simulink subsystem "April_Tag_Errors"  (R2023b)
settings: Solver=VariableStepAuto  StartTime=0.0  StopTime=10.0  RelTol=1e-3
undefined symbols (not defined in the file): AT_Tag_11_Yaw_Offset, AT_Tag_12_Yaw_Offset, AT_Tag_13_Coordinate_Y, AT_Tag_13_Yaw_Offset, AT_Tag_14_Coordinate_Y, AT_Tag_14_Yaw_Offset, AT_Tag_15_Yaw_Offset, AT_Tag_16_Yaw_Offset, AT_Tag_4_Yaw_Offset, AT_Tag_5_Coordinate_X, AT_Tag_5_Yaw_Offset, AT_Tag_6_Coordinate_X, AT_Tag_6_Yaw_Offset, AT_Tag_7_Yaw_Offset, KF_Vision_Ambiguity_Thresh
libraries: simulink x1
settings Model: Creator=ander  LastModifiedBy=ander

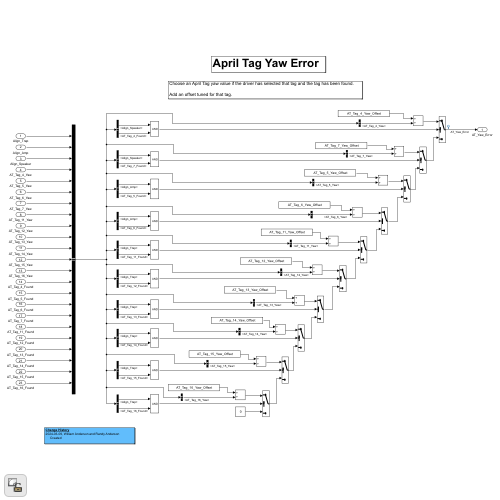
[thumbnail: Simulink's stored preview of the top-level diagram]
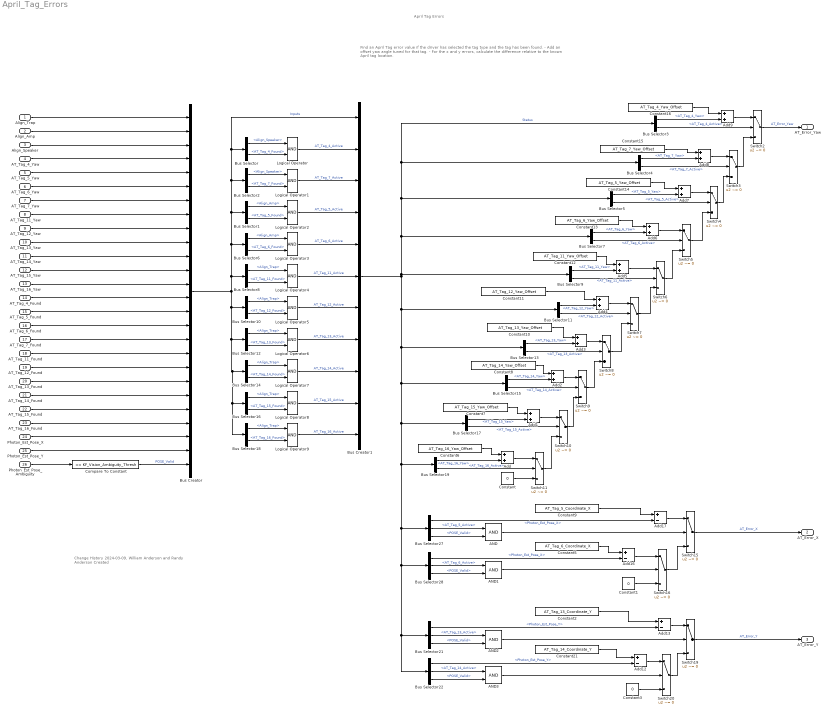
== system April_Tag_Errors ==
  note: Find an April Tag error value if the driver has selected the tag type and the tag has been found.
      | - Add an offset yaw angle tuned for that tag.
      | - For the x and y errors, calculate the difference relative to the known April tag location.
  note: Change History
      | 2024-03-09, William Anderson and Randy Anderson
      | Created
  note: April Tag Errors
  Align_Trap : Inport
  Align_Amp : Inport  Port=2
  Align_Speaker : Inport  Port=3
  AT_Tag_4_Yaw : Inport  Port=4
  AT_Tag_5_Yaw : Inport  Port=5
  AT_Tag_6_Yaw : Inport  Port=6
  AT_Tag_7_Yaw : Inport  Port=7
  AT_Tag_11_Yaw : Inport  Port=8
  AT_Tag_12_Yaw : Inport  Port=9
  AT_Tag_13_Yaw : Inport  Port=10
  AT_Tag_14_Yaw : Inport  Port=11
  AT_Tag_15_Yaw : Inport  Port=12
  AT_Tag_16_Yaw : Inport  Port=13
  AT_Tag_4_Found : Inport  Port=14
  AT_Tag_5_Found : Inport  Port=15
  AT_Tag_6_Found : Inport  Port=16
  AT_Tag_7_Found : Inport  Port=17
  AT_Tag_11_Found : Inport  Port=18
  AT_Tag_12_Found : Inport  Port=19
  AT_Tag_13_Found : Inport  Port=20
  AT_Tag_14_Found : Inport  Port=21
  AT_Tag_15_Found : Inport  Port=22
  AT_Tag_16_Found : Inport  Port=23
  Photon_Est_Pose_X : Inport  Port=24
  Photon_Est_Pose_Y : Inport  Port=25
  Photon_Est_Pose_Ambiguity : Inport  Port=26
  AND{,1..3} (4 alike) : Logic  AllPortsSameDT=off  OutDataTypeStr=boolean
  Add{,1..9} (10 alike) : Sum
  Add{12..13,16..17} (4 alike) : Sum  Inputs=+-
  Bus Creator : BusCreator  Inputs=26
  Bus Creator1 : BusCreator  Inputs=11
  Bus Selector : BusSelector  OutputSignals=Align_Speaker,AT_Tag_4_Found
  Bus Selector1 : BusSelector  OutputSignals=Align_Amp,AT_Tag_5_Found
  Bus Selector10 : BusSelector  OutputSignals=Align_Trap,AT_Tag_12_Found
  Bus Selector11 : BusSelector  OutputSignals=Inputs.AT_Tag_12_Yaw,AT_Tag_12_Active
  Bus Selector12 : BusSelector  OutputSignals=Align_Trap,AT_Tag_13_Found
  Bus Selector13 : BusSelector  OutputSignals=Inputs.AT_Tag_13_Yaw,AT_Tag_13_Active
  Bus Selector14 : BusSelector  OutputSignals=Align_Trap,AT_Tag_14_Found
  Bus Selector15 : BusSelector  OutputSignals=Inputs.AT_Tag_14_Yaw,AT_Tag_14_Active
  Bus Selector16 : BusSelector  OutputSignals=Align_Trap,AT_Tag_15_Found
  Bus Selector17 : BusSelector  OutputSignals=Inputs.AT_Tag_15_Yaw,AT_Tag_15_Active
  Bus Selector18 : BusSelector  OutputSignals=Align_Trap,AT_Tag_16_Found
  Bus Selector19 : BusSelector  OutputSignals=Inputs.AT_Tag_16_Yaw,AT_Tag_16_Active
  Bus Selector2 : BusSelector  OutputSignals=Align_Speaker,AT_Tag_7_Found
  Bus Selector21 : BusSelector  OutputSignals=Inputs.Photon_Est_Pose_Y,AT_Tag_13_Active,Inputs.POSE_Valid
  Bus Selector22 : BusSelector  OutputSignals=Inputs.Photon_Est_Pose_Y,AT_Tag_14_Active,Inputs.POSE_Valid
  Bus Selector27 : BusSelector  OutputSignals=Inputs.Photon_Est_Pose_X,AT_Tag_5_Active,Inputs.POSE_Valid
  Bus Selector28 : BusSelector  OutputSignals=Inputs.Photon_Est_Pose_X,AT_Tag_6_Active,Inputs.POSE_Valid
  Bus Selector3 : BusSelector  OutputSignals=Inputs.AT_Tag_4_Yaw,AT_Tag_4_Active
  Bus Selector4 : BusSelector  OutputSignals=Inputs.AT_Tag_7_Yaw,AT_Tag_7_Active
  Bus Selector5 : BusSelector  OutputSignals=Inputs.AT_Tag_5_Yaw,AT_Tag_5_Active
  Bus Selector6 : BusSelector  OutputSignals=Align_Amp,AT_Tag_6_Found
  Bus Selector7 : BusSelector  OutputSignals=Inputs.AT_Tag_6_Yaw,AT_Tag_6_Active
  Bus Selector8 : BusSelector  OutputSignals=Align_Trap,AT_Tag_11_Found
  Bus Selector9 : BusSelector  OutputSignals=Inputs.AT_Tag_11_Yaw,AT_Tag_11_Active
  Compare To Constant : simulink/Logic and Bit Operations/Compare To Constant  relop=<=  const=KF_Vision_Ambiguity_Thresh  OutDataTypeStr=boolean
  Constant : Constant  Value=0
  Constant1 : Constant  Value=0
  Constant10 : Constant  Value=AT_Tag_13_Yaw_Offset
  Constant11 : Constant  Value=AT_Tag_12_Yaw_Offset
  Constant12 : Constant  Value=AT_Tag_11_Yaw_Offset
  Constant13 : Constant  Value=AT_Tag_6_Yaw_Offset
  Constant14 : Constant  Value=AT_Tag_5_Yaw_Offset
  Constant15 : Constant  Value=AT_Tag_7_Yaw_Offset
  Constant16 : Constant  Value=AT_Tag_4_Yaw_Offset
  Constant2 : Constant  Value=AT_Tag_13_Coordinate_Y
  Constant21 : Constant  Value=AT_Tag_14_Coordinate_Y
  Constant3 : Constant  Value=0
  Constant5 : Constant  Value=AT_Tag_6_Coordinate_X
  Constant6 : Constant  Value=AT_Tag_16_Yaw_Offset
  Constant7 : Constant  Value=AT_Tag_15_Yaw_Offset
  Constant8 : Constant  Value=AT_Tag_14_Yaw_Offset
  Constant9 : Constant  Value=AT_Tag_5_Coordinate_X
  Logical Operator{,1..9} (10 alike) : Logic  AllPortsSameDT=off  OutDataTypeStr=boolean
  Switch{2..11,15..16,19..20} (14 alike) : Switch  Criteria=u2 ~= 0  SaturateOnIntegerOverflow=off  InputSameDT=off
  AT_Error_Yaw : Outport
  AT_Error_X : Outport  Port=2
  AT_Error_Y : Outport  Port=3
  wires:
  Switch19/1 -> AT_Error_Y/1  "AT_Error_Y"
  Switch15/1 -> AT_Error_X/1  "AT_Error_X"
  Constant3/1 -> Switch20/3
  Constant1/1 -> Switch16/3
  Constant5/1 -> Add16/1
  Constant2/1 -> Add13/1
  Add13/1 -> Switch19/1
  Switch20/1 -> Switch19/3
  Add16/1 -> Switch16/1
  Bus Creator1/1 -> Bus Selector13/1, Bus Selector15/1, Bus Selector17/1, Bus Selector27/1, Bus Selector28/1, Bus Selector21/1, Bus Selector22/1, Bus Selector19/1, Bus Selector11/1, Bus Selector3/1, Bus Selector4/1, Bus Selector5/1, Bus Selector7/1, Bus Selector9/1  "Status"
  Add17/1 -> Switch15/1
  Constant21/1 -> Add12/1
  Constant9/1 -> Add17/1
  Add12/1 -> Switch20/1
  Switch16/1 -> Switch15/3
  Bus Selector19/2 -> Switch11/2  "<AT_Tag_16_Active>"
  Bus Selector17/2 -> Switch10/2  "<AT_Tag_15_Active>"
  Bus Selector15/2 -> Switch9/2  "<AT_Tag_14_Active>"
  Bus Selector13/2 -> Switch8/2  "<AT_Tag_13_Active>"
  Bus Selector11/2 -> Switch7/2  "<AT_Tag_12_Active>"
  Bus Selector9/2 -> Switch6/2  "<AT_Tag_11_Active>"
  Bus Selector7/2 -> Switch5/2  "<AT_Tag_6_Active>"
  Bus Selector5/2 -> Switch4/2  "<AT_Tag_5_Active>"
  Bus Selector4/2 -> Switch3/2  "<AT_Tag_7_Active>"
  Bus Selector3/2 -> Switch2/2  "<AT_Tag_4_Active>"
  Logical Operator9/1 -> Bus Creator1/11  "AT_Tag_16_Active"
  Logical Operator8/1 -> Bus Creator1/10  "AT_Tag_15_Active"
  Logical Operator7/1 -> Bus Creator1/9  "AT_Tag_14_Active"
  Logical Operator6/1 -> Bus Creator1/8  "AT_Tag_13_Active"
  Logical Operator5/1 -> Bus Creator1/7  "AT_Tag_12_Active"
  Logical Operator4/1 -> Bus Creator1/6  "AT_Tag_11_Active"
  Logical Operator3/1 -> Bus Creator1/5  "AT_Tag_6_Active"
  Logical Operator2/1 -> Bus Creator1/4  "AT_Tag_5_Active"
  Logical Operator1/1 -> Bus Creator1/3  "AT_Tag_7_Active"
  Logical Operator/1 -> Bus Creator1/2  "AT_Tag_4_Active"
  AT_Tag_16_Found/1 -> Bus Creator/23
  AT_Tag_13_Found/1 -> Bus Creator/20
  AT_Tag_12_Found/1 -> Bus Creator/19
  AT_Tag_6_Found/1 -> Bus Creator/16
  AT_Tag_13_Yaw/1 -> Bus Creator/10
  AT_Tag_14_Yaw/1 -> Bus Creator/11
  AT_Tag_4_Found/1 -> Bus Creator/14
  AT_Tag_5_Found/1 -> Bus Creator/15
  AT_Tag_16_Yaw/1 -> Bus Creator/13
  AT_Tag_12_Yaw/1 -> Bus Creator/9
  AT_Tag_5_Yaw/1 -> Bus Creator/5
  AT_Tag_4_Yaw/1 -> Bus Creator/4
  Align_Amp/1 -> Bus Creator/2
  Align_Trap/1 -> Bus Creator/1
  AT_Tag_6_Yaw/1 -> Bus Creator/6
  AT_Tag_15_Yaw/1 -> Bus Creator/12
  Bus Selector7/1 -> Add6/2  "<AT_Tag_6_Yaw>"
  Add7/1 -> Switch4/1
  Constant8/1 -> Add2/1
  Constant7/1 -> Add1/1
  Bus Selector9/1 -> Add5/2  "<AT_Tag_11_Yaw>"
  Bus Selector19/1 -> Add/2  "<AT_Tag_16_Yaw>"
  Add1/1 -> Switch10/1
  Add6/1 -> Switch5/1
  Bus Selector5/1 -> Add7/2  "<AT_Tag_5_Yaw>"
  Bus Selector17/1 -> Add1/2  "<AT_Tag_15_Yaw>"
  AT_Tag_14_Found/1 -> Bus Creator/21
  Bus Selector14/1 -> Logical Operator7/1  "<Align_Trap>"
  Bus Selector14/2 -> Logical Operator7/2  "<AT_Tag_14_Found>"
  AT_Tag_7_Yaw/1 -> Bus Creator/7
  Constant/1 -> Switch11/3
  Bus Selector15/1 -> Add2/2  "<AT_Tag_14_Yaw>"
  Bus Selector1/1 -> Logical Operator2/1  "<Align_Amp>"
  AT_Tag_11_Found/1 -> Bus Creator/18
  Constant12/1 -> Add5/1
  Constant15/1 -> Add8/1
  Bus Selector10/2 -> Logical Operator5/2  "<AT_Tag_12_Found>"
  Switch7/1 -> Switch6/3
  Constant10/1 -> Add3/1
  Bus Selector2/1 -> Logical Operator1/1  "<Align_Speaker>"
  Bus Selector8/1 -> Logical Operator4/1  "<Align_Trap>"
  Switch10/1 -> Switch9/3
  Switch3/1 -> Switch2/3
  Bus Selector12/2 -> Logical Operator6/2  "<AT_Tag_13_Found>"
  Switch5/1 -> Switch4/3
  Constant14/1 -> Add7/1
  Bus Selector1/2 -> Logical Operator2/2  "<AT_Tag_5_Found>"
  Constant16/1 -> Add9/1
  Bus Selector6/1 -> Logical Operator3/1  "<Align_Amp>"
  Bus Selector18/2 -> Logical Operator9/2  "<AT_Tag_16_Found>"
  Bus Selector3/1 -> Add9/2  "<AT_Tag_4_Yaw>"
  Bus Selector16/2 -> Logical Operator8/2  "<AT_Tag_15_Found>"
  Bus Selector12/1 -> Logical Operator6/1  "<Align_Trap>"
  Bus Selector4/1 -> Add8/2  "<AT_Tag_7_Yaw>"
  Add9/1 -> Switch2/1
  AT_Tag_7_Found/1 -> Bus Creator/17
  Align_Speaker/1 -> Bus Creator/3
  Bus Selector8/2 -> Logical Operator4/2  "<AT_Tag_11_Found>"
  Bus Selector2/2 -> Logical Operator1/2  "<AT_Tag_7_Found>"
  Add/1 -> Switch11/1
  Bus Selector11/1 -> Add4/2  "<AT_Tag_12_Yaw>"
  Switch2/1 -> AT_Error_Yaw/1  "AT_Error_Yaw"
  Add8/1 -> Switch3/1
  Bus Selector10/1 -> Logical Operator5/1  "<Align_Trap>"
  Add2/1 -> Switch9/1
  Switch6/1 -> Switch5/3
  Bus Selector13/1 -> Add3/2  "<AT_Tag_13_Yaw>"
  Switch11/1 -> Switch10/3
  Bus Selector/2 -> Logical Operator/2  "<AT_Tag_4_Found>"
  Bus Selector6/2 -> Logical Operator3/2  "<AT_Tag_6_Found>"
  Switch9/1 -> Switch8/3
  Add5/1 -> Switch6/1
  Bus Selector/1 -> Logical Operator/1  "<Align_Speaker>"
  Bus Selector16/1 -> Logical Operator8/1  "<Align_Trap>"
  Bus Creator/1 -> Bus Creator1/1, Bus Selector/1, Bus Selector2/1, Bus Selector1/1, Bus Selector6/1, Bus Selector8/1, Bus Selector10/1, Bus Selector18/1, Bus Selector16/1, Bus Selector14/1, Bus Selector12/1  "Inputs"
  Constant11/1 -> Add4/1
  Switch4/1 -> Switch3/3
  Constant13/1 -> Add6/1
  AT_Tag_15_Found/1 -> Bus Creator/22
  Bus Selector18/1 -> Logical Operator9/1  "<Align_Trap>"
  Switch8/1 -> Switch7/3
  AT_Tag_11_Yaw/1 -> Bus Creator/8
  Constant6/1 -> Add/1
  Add3/1 -> Switch8/1
  Add4/1 -> Switch7/1
  Photon_Est_Pose_X/1 -> Bus Creator/24
  Photon_Est_Pose_Y/1 -> Bus Creator/25
  Photon_Est_Pose_Ambiguity/1 -> Compare To Constant/1
  Bus Selector27/1 -> Add17/2  "<Photon_Est_Pose_X>"
  Bus Selector27/2 -> AND/1  "<AT_Tag_5_Active>"
  AND/1 -> Switch15/2
  Compare To Constant/1 -> Bus Creator/26  "POSE_Valid"
  Bus Selector27/3 -> AND/2  "<POSE_Valid>"
  Bus Selector28/1 -> Add16/2  "<Photon_Est_Pose_X>"
  Bus Selector28/2 -> AND1/1  "<AT_Tag_6_Active>"
  Bus Selector28/3 -> AND1/2  "<POSE_Valid>"
  AND1/1 -> Switch16/2
  Bus Selector21/1 -> Add13/2  "<Photon_Est_Pose_Y>"
  Bus Selector21/2 -> AND2/1  "<AT_Tag_13_Active>"
  Bus Selector21/3 -> AND2/2  "<POSE_Valid>"
  AND2/1 -> Switch19/2
  Bus Selector22/1 -> Add12/2  "<Photon_Est_Pose_Y>"
  Bus Selector22/2 -> AND3/1  "<AT_Tag_14_Active>"
  Bus Selector22/3 -> AND3/2  "<POSE_Valid>"
  AND3/1 -> Switch20/2
